simulink model "ResetZeroPosition"  (R2022a)
settings: Solver=VariableStepAuto  StartTime=0.0  StopTime=10.0  RelTol=1e-3
settings Model: Creator=randolf  LastModifiedBy=randolf

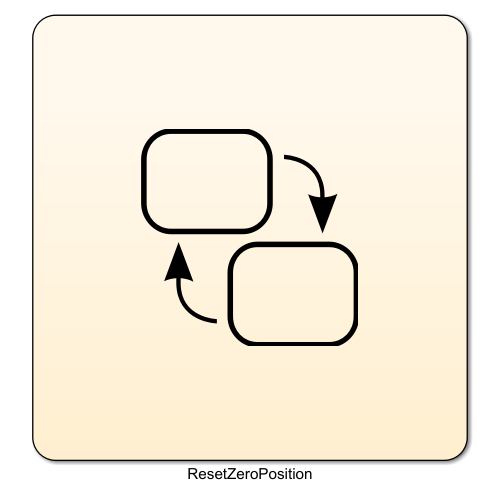
[thumbnail: Simulink's stored preview of the top-level diagram]
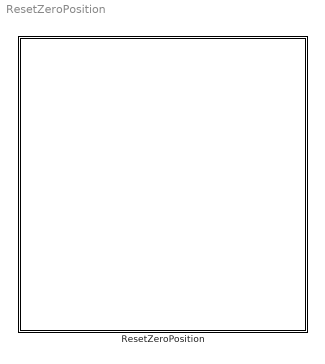
== system ResetZeroPosition ==
  ResetZeroPosition : Stateflow chart  TreatAsAtomicUnit=on

== stateflow chart ResetZeroPosition/ResetZeroPosition ==
  state HoldOn
  state ChaseBackZeroPosition
  state ExecutionMovement
  (default) -> HoldOn
  ChaseBackZeroPosition -> HoldOn
  HoldOn -> ExecutionMovement
  ExecutionMovement -> ChaseBackZeroPosition
